simulink model "simulation_scheme_vel"  (R2021b)
settings: Solver=FixedStepAuto  StartTime=0.0  StopTime=simulation.stop_time  FixedStep=simulation.step_size  RelTol=1e-5
PreLoadFcn:
  | % initialize variables
  | initializeUnicycleModel;
undefined symbols (not defined in the file): camera, controller, obstacle, park, scheduler, simulation, tracking, unicycle
settings Model: Creator=beniamino  LastModifiedBy=gioel
settings SolverCC: AlgebraicLoopSolver=TrustRegion
settings DataIOCC: InitialState=cartesianInitialStates  SaveFormat=Structure

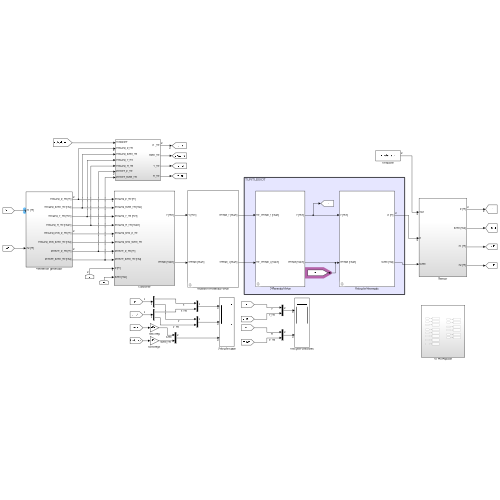
[thumbnail: Simulink's stored preview of the top-level diagram]
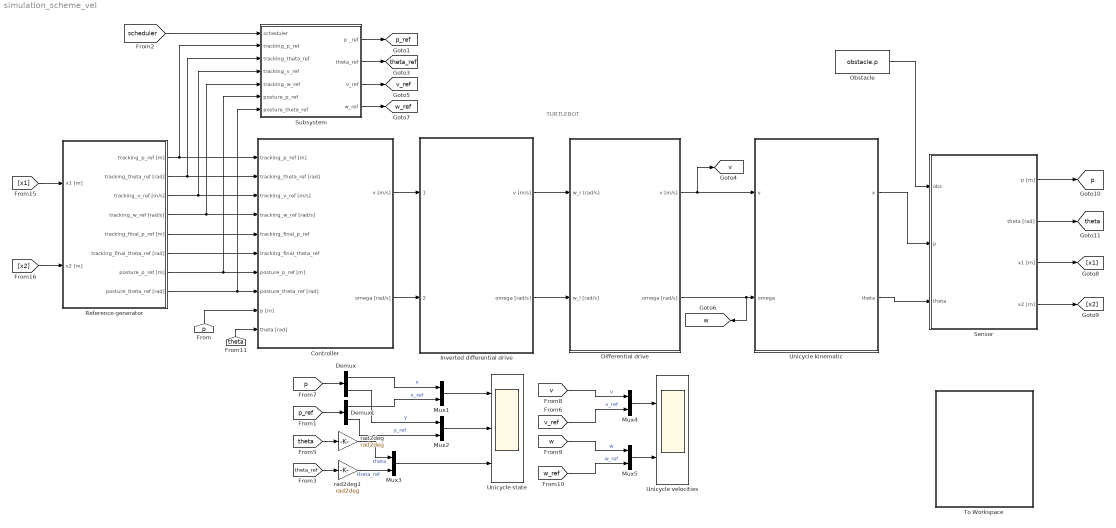
== system simulation_scheme_vel ==
  note: TURTLEBOT
  Controller : Subsystem
  Demux : Demux  Outputs=2
  Demux1 : Demux  Outputs=2
  Differential drive : Subsystem  mask(Differential drive for a unicycle){r=unicycle.diffDrive.r, d=unicycle.diffDrive.d, wheelDyEn=on, Tc=unicycle.diffDrive.Td, wheelsSpeedUpperLimit=unicycle.diffDrive.omegaWheelMax, wheelsSpeedLowerLimit=unicycle.diffDrive.omegaWheelMin}
      mask prompts: r "wheel radius"; d "interaxis lenght"; wheelDyEn "l.p.f. enable"; Tc "time constant [s]"; wheelsSpeedUpperLimit "max wheel speed  [rad/s]"; wheelsSpeedLowerLimit "min wheel speed [rad/s]"
      mask help:
      | Model of a differential drive.
      | It takes as input the derired wheel velocities and converts them to the corresponding driving velocity and stearing velocity.
      | Wheels dynamics can be taken into accont, along with output saturation.
      mask Help:
      | author: Beniamino Pozzan
      | email: beniamino.pozzan@phd.unipd.it
      mask Callback wheelDyEn:
      | % get the enable parameter
      | wheelDyEnStatus = get_param(gcb,'wheelDyEn');
      | enableStatus = get_param(gcb,'MaskEnables');
      | % if it is true, make Tc enabled
      | if strcmp(wheelDyEnStatus,'on')
      |     enableStatus{4}='on';
      | else
      |     enableStatus{4}='off';
      | end
      | set_param(gcb,'MaskEnables',enableStatus)
      mask TypeOptions wheelsSpeedUpperLimit: w_l saturator/UpperLimit | w_r saturator/UpperLimit
      mask TypeOptions wheelsSpeedLowerLimit: w_l saturator/LowerLimit | w_r saturator/LowerLimit
      mask DialogControl wheelDy Prompt: wheel dynamics
  Inverted differential drive : Subsystem  mask(Inverted Differential drive for a unicycle){r=unicycle.diffDrive.r, d=unicycle.diffDrive.d}
      mask prompts: r "wheel radius"; d "interaxis lenght"
      mask help:
      | Inverted differential drive for a unicycle.
      | Provided the desired driving and stearing velocities, it computes the corresponding wheel velocities.
  Mux{1..5} (5 alike) : Mux  Inputs=2
  Obstacle : Constant  Value=obstacle.p
  Reference generator : Subsystem
  Sensor : Subsystem
  Subsystem : Subsystem
  To Workspace : Subsystem
  Unicycle kinematic : Subsystem  mask(Unicycle Kinematic Model){x0=unicycle.ic.x, y0=unicycle.ic.y, theta0=unicycle.ic.theta}
      mask prompts: x0 "x_0"; y0 "y_0"; theta0 "theta_0"
      mask help: kinematic model of a unicyle.
  Unicycle state : Scope  NumInputPorts=3
  Unicycle velocities : Scope  NumInputPorts=2
  rad2deg : Gain  Gain=rad2deg
  rad2deg1 : Gain  Gain=rad2deg
  tag scope: p=global, p_ref=global, theta=global, theta_ref=global, v=global, v_ref=global, w=global, w_ref=global
  wires:
  Inverted differential drive/1(v [m/s]) -> Differential drive/1(w_r [rad/s])
  Inverted differential drive/2(omega [rad/s]) -> Differential drive/2(w_l [rad/s])
  Differential drive/1(v [m/s]) -> Unicycle kinematic/1(v), [v]
  Differential drive/2(omega [rad/s]) -> [w], Unicycle kinematic/2(omega)
  Unicycle kinematic/1(x) -> Sensor/2(p)
  Unicycle kinematic/2(theta) -> Sensor/3(theta)
  [p] -> Demux/1
  [p_ref] -> Demux1/1
  Mux1/1 -> Unicycle state/1
  Mux2/1 -> Unicycle state/2
  Demux/1 -> Mux1/1  "x"
  Demux1/1 -> Mux1/2  "x_ref"
  Demux/2 -> Mux2/1  "y"
  Demux1/2 -> Mux2/2  "y_ref"
  [theta_ref] -> rad2deg1/1
  Mux4/1 -> Unicycle velocities/1
  Mux5/1 -> Unicycle velocities/2
  [v] -> Mux4/1  "v"
  [v_ref] -> Mux4/2  "v_ref"
  [w] -> Mux5/1  "w"
  [w_ref] -> Mux5/2  "w_ref"
  [theta] -> Controller/10(theta [rad])
  Controller/1(v [m/s]) -> Inverted differential drive/1(1)
  Controller/2(omega [rad/s]) -> Inverted differential drive/2(2)
  Reference generator/1(tracking_p_ref [m]) -> Subsystem/2(tracking_p_ref), Controller/1(tracking_p_ref [m])
  Reference generator/4(tracking_w_ref [rad/s]) -> Subsystem/5(tracking_w_ref), Controller/4(tracking_w_ref [rad/s])
  Reference generator/2(tracking_theta_ref [rad]) -> Subsystem/3(tracking_theta_ref), Controller/2(tracking_theta_ref [rad])
  Reference generator/5(tracking_final_p_ref [m]) -> Controller/5(tracking_final_p_ref)
  Reference generator/6(tracking_final_theta_ref [rad]) -> Controller/6(tracking_final_theta_ref)
  Reference generator/7(posture_p_ref [m]) -> Subsystem/6(posture_p_ref), Controller/7(posture_p_ref [m])
  Reference generator/8(posture_theta_ref [rad]) -> Subsystem/7(posture_theta_ref), Controller/8(posture_theta_ref [rad])
  Reference generator/3(tracking_v_ref [m/s]) -> Subsystem/4(tracking_v_ref), Controller/3(tracking_v_ref [m/s])
  Mux3/1 -> Unicycle state/3
  Sensor/1(p [m]) -> [p]
  Sensor/2(theta [rad]) -> [theta]
  Sensor/3(x1 [m]) -> [x1]
  Sensor/4(x2 [m]) -> [x2]
  Obstacle/1 -> Sensor/1(obs)
  [x1] -> Reference generator/1(x1 [m])
  [x2] -> Reference generator/2(x2 [m])
  [p] -> Controller/9(p [m])
  [theta] -> rad2deg/1
  rad2deg/1 -> Mux3/1  "theta"
  rad2deg1/1 -> Mux3/2  "theta_ref"
  Subsystem/1(p _ref) -> [p_ref]
  Subsystem/2(theta_ref) -> [theta_ref]
  Subsystem/3(v_ref) -> [v_ref]
  Subsystem/4(w_ref) -> [w_ref]
  [scheduler] -> Subsystem/1(scheduler)

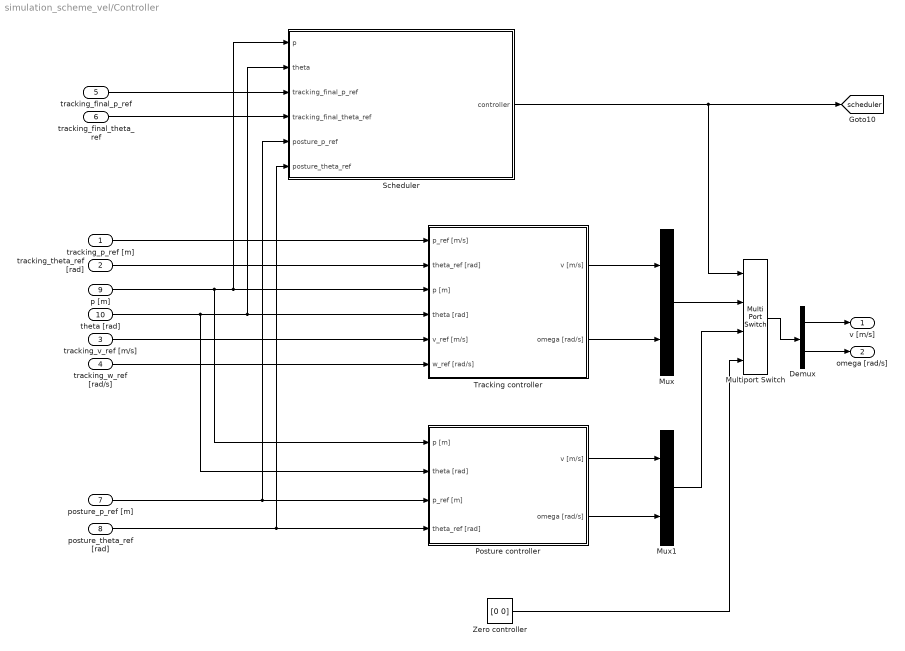
== system simulation_scheme_vel/Controller ==
  tracking_p_ref [m] : Inport
  tracking_theta_ref [rad] : Inport  Port=2
  tracking_v_ref [m/s] : Inport  Port=3
  tracking_w_ref [rad/s] : Inport  Port=4
  tracking_final_p_ref : Inport  Port=5
  tracking_final_theta_ref : Inport  Port=6
  posture_p_ref [m] : Inport  Port=7
  posture_theta_ref [rad] : Inport  Port=8
  p [m] : Inport  Port=9
  theta [rad] : Inport  Port=10
  Demux : Demux  Outputs=2
  Multiport Switch : MultiPortSwitch
  Mux : Mux  Inputs=2
  Mux1 : Mux  Inputs=2
  Posture controller : Subsystem
  Scheduler : MATLAB Function  TreatAsAtomicUnit=on
  Tracking controller : Subsystem
  Zero controller : Constant  Value=[0 0]
  v [m/s] : Outport
  omega [rad/s] : Outport  Port=2
  tag scope: scheduler=global
  wires:
  Multiport Switch/1 -> Demux/1
  Tracking controller/1(v [m/s]) -> Mux/1
  Tracking controller/2(omega [rad/s]) -> Mux/2
  Demux/2 -> omega [rad/s]/1
  Demux/1 -> v [m/s]/1
  Mux/1 -> Multiport Switch/2
  tracking_p_ref [m]/1 -> Tracking controller/1(p_ref [m/s])
  tracking_theta_ref [rad]/1 -> Tracking controller/2(theta_ref [rad])
  p [m]/1 -> Posture controller/1(p [m]), Tracking controller/3(p [m]), Scheduler/1(p)
  Zero controller/1 -> Multiport Switch/4
  Mux1/1 -> Multiport Switch/3
  Posture controller/2(omega [rad/s]) -> Mux1/2
  Posture controller/1(v [m/s]) -> Mux1/1
  Scheduler/1(controller) -> [scheduler], Multiport Switch/1
  theta [rad]/1 -> Posture controller/2(theta [rad]), Tracking controller/4(theta [rad]), Scheduler/2(theta)
  posture_p_ref [m]/1 -> Posture controller/3(p_ref [m]), Scheduler/5(posture_p_ref)
  posture_theta_ref [rad]/1 -> Scheduler/6(posture_theta_ref), Posture controller/4(theta_ref [rad])
  tracking_final_p_ref/1 -> Scheduler/3(tracking_final_p_ref)
  tracking_final_theta_ref/1 -> Scheduler/4(tracking_final_theta_ref)
  tracking_v_ref [m/s]/1 -> Tracking controller/5(v_ref [m/s])
  tracking_w_ref [rad/s]/1 -> Tracking controller/6(w_ref [rad/s])

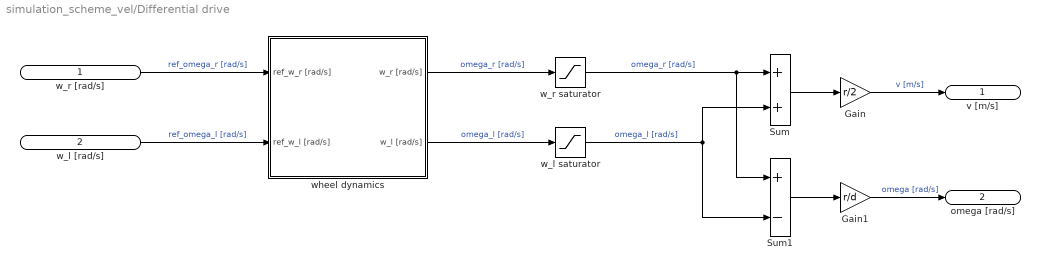
== system simulation_scheme_vel/Differential drive ==
  w_r [rad/s] : Inport  Unit=rad/s
  w_l [rad/s] : Inport  Port=2  Unit=rad/s
  Gain : Gain  Gain=r/2
  Gain1 : Gain  Gain=r/d
  Sum : Sum
  Sum1 : Sum  Inputs=+-
  w_l saturator : Saturate  UpperLimit=wheelsSpeedUpperLimit  LowerLimit=wheelsSpeedLowerLimit
  w_r saturator : Saturate  UpperLimit=wheelsSpeedUpperLimit  LowerLimit=wheelsSpeedLowerLimit
  wheel dynamics : Subsystem  Variant=on
  v [m/s] : Outport  Unit=m/s
  omega [rad/s] : Outport  Port=2  Unit=rad/s
  wires:
  w_l saturator/1 -> Sum1/2, Sum/2  "omega_l [rad/s]"
  w_r saturator/1 -> Sum1/1, Sum/1  "omega_r [rad/s]"
  Gain1/1 -> omega [rad/s]/1  "omega [rad/s]"
  Sum1/1 -> Gain1/1
  Gain/1 -> v [m/s]/1  "v [m/s]"
  Sum/1 -> Gain/1
  w_r [rad/s]/1 -> wheel dynamics/1(ref_w_r [rad/s])  "ref_omega_r [rad/s]"
  w_l [rad/s]/1 -> wheel dynamics/2(ref_w_l [rad/s])  "ref_omega_l [rad/s]"
  wheel dynamics/1(w_r [rad/s]) -> w_r saturator/1  "omega_r [rad/s]"
  wheel dynamics/2(w_l [rad/s]) -> w_l saturator/1  "omega_l [rad/s]"

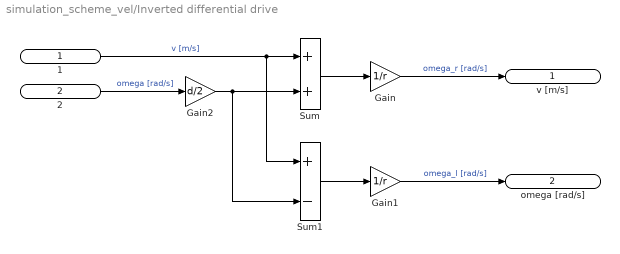
== system simulation_scheme_vel/Inverted differential drive ==
  1 : Inport  Unit=m/s
  2 : Inport  Port=2  Unit=rad/s
  Gain : Gain  Gain=1/r
  Gain1 : Gain  Gain=1/r
  Gain2 : Gain  Gain=d/2
  Sum : Sum
  Sum1 : Sum  Inputs=+-
  v [m/s] : Outport  Unit=rad/s
  omega [rad/s] : Outport  Port=2  Unit=rad/s
  wires:
  Gain2/1 -> Sum1/2, Sum/2
  Sum/1 -> Gain/1
  Gain/1 -> v [m/s]/1  "omega_r [rad/s]"
  Sum1/1 -> Gain1/1
  Gain1/1 -> omega [rad/s]/1  "omega_l [rad/s]"
  1/1 -> Sum1/1, Sum/1  "v [m/s]"
  2/1 -> Gain2/1  "omega [rad/s]"

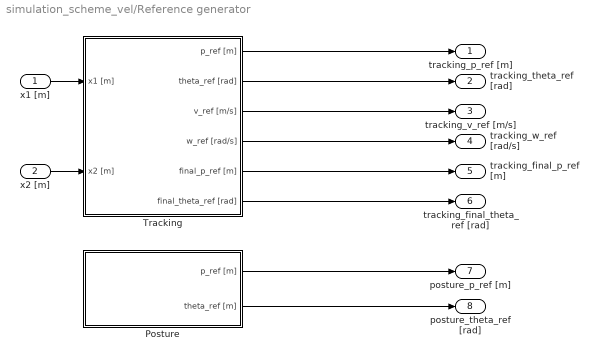
== system simulation_scheme_vel/Reference generator ==
  x1 [m] : Inport
  x2 [m] : Inport  Port=2
  Posture : Subsystem
  Tracking : Subsystem
  tracking_p_ref [m] : Outport
  tracking_theta_ref [rad] : Outport  Port=2
  tracking_v_ref [m/s] : Outport  Port=3
  tracking_w_ref [rad/s] : Outport  Port=4
  tracking_final_p_ref [m] : Outport  Port=5
  tracking_final_theta_ref [rad] : Outport  Port=6
  posture_p_ref [m] : Outport  Port=7
  posture_theta_ref [rad] : Outport  Port=8
  wires:
  Tracking/4(w_ref [rad/s]) -> tracking_w_ref [rad/s]/1
  Tracking/3(v_ref [m/s]) -> tracking_v_ref [m/s]/1
  Posture/1(p_ref [m]) -> posture_p_ref [m]/1
  Tracking/5(final_p_ref [m]) -> tracking_final_p_ref [m]/1
  Tracking/2(theta_ref [rad]) -> tracking_theta_ref [rad]/1
  Tracking/6(final_theta_ref [rad]) -> tracking_final_theta_ref [rad]/1
  Tracking/1(p_ref [m]) -> tracking_p_ref [m]/1
  Posture/2(theta_ref [m]) -> posture_theta_ref [rad]/1
  x2 [m]/1 -> Tracking/2(x2 [m])
  x1 [m]/1 -> Tracking/1(x1 [m])

== system simulation_scheme_vel/Sensor ==
  obs : Inport
  p : Inport  Port=2
  theta : Inport  Port=3
  Demux : Demux  Outputs=2
  camera : MATLAB Function  TreatAsAtomicUnit=on
  p [m] : Outport
  theta [rad] : Outport  Port=2
  x1 [m] : Outport  Port=3
  x2 [m] : Outport  Port=4
  wires:
  camera/2(x2) -> x2 [m]/1
  camera/1(x1) -> x1 [m]/1
  theta/1 -> camera/3(theta), theta [rad]/1
  obs/1 -> camera/4(obs_W)
  p/1 -> Demux/1, p [m]/1
  Demux/1 -> camera/1(x_pos)
  Demux/2 -> camera/2(y_pos)

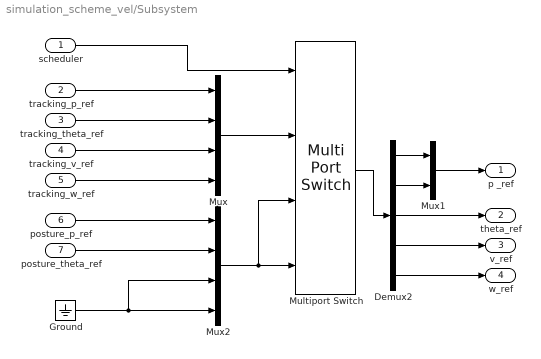
== system simulation_scheme_vel/Subsystem ==
  scheduler : Inport
  tracking_p_ref : Inport  Port=2
  tracking_theta_ref : Inport  Port=3
  tracking_v_ref : Inport  Port=4
  tracking_w_ref : Inport  Port=5
  posture_p_ref : Inport  Port=6
  posture_theta_ref : Inport  Port=7
  Demux2 : Demux  Outputs=5
  Ground : Ground
  Multiport Switch : MultiPortSwitch
  Mux : Mux
  Mux1 : Mux  Inputs=2
  Mux2 : Mux
  p _ref : Outport
  theta_ref : Outport  Port=2
  v_ref : Outport  Port=3
  w_ref : Outport  Port=4
  wires:
  tracking_theta_ref/1 -> Mux/2
  scheduler/1 -> Multiport Switch/1
  tracking_p_ref/1 -> Mux/1
  Multiport Switch/1 -> Demux2/1
  Mux/1 -> Multiport Switch/2
  Ground/1 -> Mux2/3, Mux2/4
  tracking_v_ref/1 -> Mux/3
  tracking_w_ref/1 -> Mux/4
  Mux2/1 -> Multiport Switch/3, Multiport Switch/4
  posture_p_ref/1 -> Mux2/1
  posture_theta_ref/1 -> Mux2/2
  Demux2/1 -> Mux1/1
  Demux2/2 -> Mux1/2
  Mux1/1 -> p _ref/1
  Demux2/3 -> theta_ref/1
  Demux2/4 -> v_ref/1
  Demux2/5 -> w_ref/1

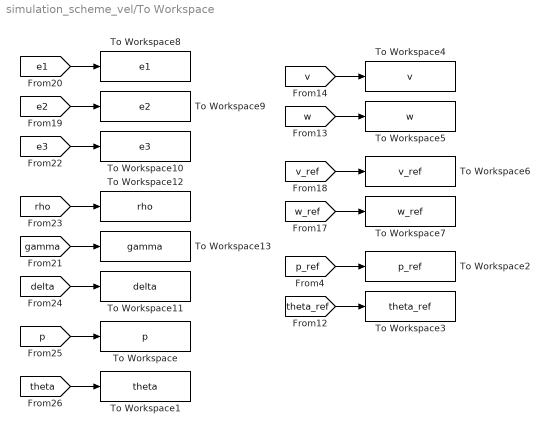
== system simulation_scheme_vel/To Workspace ==
  To Workspace : ToWorkspace  VariableName=p  SaveFormat=Timeseries  SampleTime=-1
  To Workspace1 : ToWorkspace  VariableName=theta  SaveFormat=Timeseries  SampleTime=-1
  To Workspace10 : ToWorkspace  VariableName=e3  SaveFormat=Timeseries  SampleTime=-1
  To Workspace11 : ToWorkspace  VariableName=delta  SaveFormat=Timeseries  SampleTime=-1
  To Workspace12 : ToWorkspace  VariableName=rho  SaveFormat=Timeseries  SampleTime=-1
  To Workspace13 : ToWorkspace  VariableName=gamma  SaveFormat=Timeseries  SampleTime=-1
  To Workspace2 : ToWorkspace  VariableName=p_ref  SaveFormat=Timeseries  SampleTime=-1
  To Workspace3 : ToWorkspace  VariableName=theta_ref  SaveFormat=Timeseries  SampleTime=-1
  To Workspace4 : ToWorkspace  VariableName=v  SaveFormat=Timeseries  SampleTime=-1
  To Workspace5 : ToWorkspace  VariableName=w  SaveFormat=Timeseries  SampleTime=-1
  To Workspace6 : ToWorkspace  VariableName=v_ref  SaveFormat=Timeseries  SampleTime=-1
  To Workspace7 : ToWorkspace  VariableName=w_ref  SaveFormat=Timeseries  SampleTime=-1
  To Workspace8 : ToWorkspace  VariableName=e1  SaveFormat=Timeseries  SampleTime=-1
  To Workspace9 : ToWorkspace  VariableName=e2  SaveFormat=Timeseries  SampleTime=-1
  wires:
  [v_ref] -> To Workspace6/1
  [w_ref] -> To Workspace7/1
  [theta] -> To Workspace1/1
  [e1] -> To Workspace8/1
  [v] -> To Workspace4/1
  [e2] -> To Workspace9/1
  [delta] -> To Workspace11/1
  [gamma] -> To Workspace13/1
  [e3] -> To Workspace10/1
  [w] -> To Workspace5/1
  [rho] -> To Workspace12/1
  [p_ref] -> To Workspace2/1
  [theta_ref] -> To Workspace3/1
  [p] -> To Workspace/1

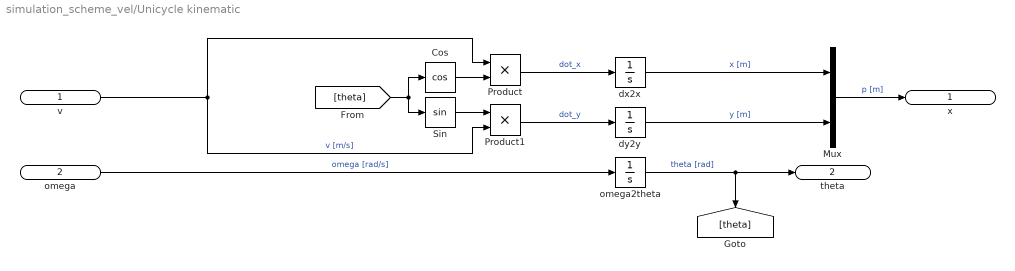
== system simulation_scheme_vel/Unicycle kinematic ==
  v : Inport  PortDimensions=1
  omega : Inport  Port=2  PortDimensions=1
  Cos : Trigonometry  Operator=cos
  Mux : Mux  Inputs=2
  Product : Product
  Product1 : Product
  Sin : Trigonometry
  dx2x : Integrator  InitialCondition=x0  ContinuousStateAttributes='pos_x'
  dy2y : Integrator  InitialCondition=y0  ContinuousStateAttributes='pos_y'
  omega2theta : Integrator  InitialCondition=theta0  ContinuousStateAttributes='theta'
  x : Outport  PortDimensions=2
  theta : Outport  Port=2  PortDimensions=1
  wires:
  Product1/1 -> dy2y/1  "dot_y"
  [theta] -> Sin/1, Cos/1
  v/1 -> Product/1, Product1/2  "v [m/s]"
  omega2theta/1 -> [theta], theta/1  "theta [rad]"
  omega/1 -> omega2theta/1  "omega [rad/s]"
  dy2y/1 -> Mux/2  "y [m]"
  Cos/1 -> Product/2
  dx2x/1 -> Mux/1  "x [m]"
  Sin/1 -> Product1/1
  Product/1 -> dx2x/1  "dot_x"
  Mux/1 -> x/1  "p [m]"

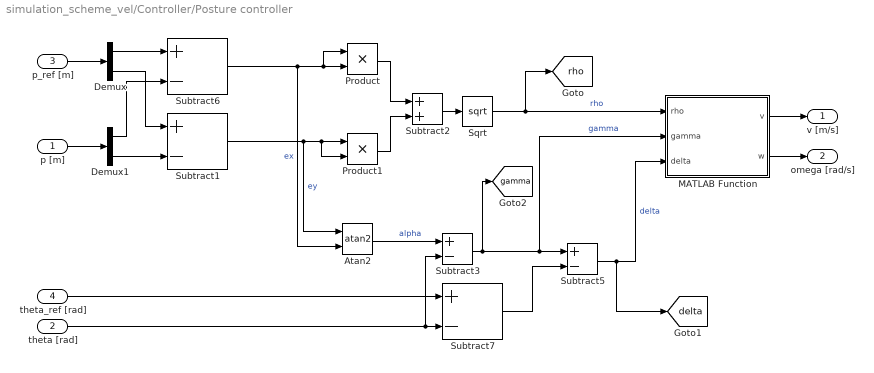
== system simulation_scheme_vel/Controller/Posture controller ==
  p [m] : Inport
  theta [rad] : Inport  Port=2
  p_ref [m] : Inport  Port=3
  theta_ref [rad] : Inport  Port=4
  Atan2 : Trigonometry  Operator=atan2
  Demux : Demux  Outputs=2
  Demux1 : Demux  Outputs=2
  MATLAB Function : MATLAB Function  TreatAsAtomicUnit=on
  Product : Product
  Product1 : Product
  Sqrt : Sqrt  SaturateOnIntegerOverflow=on
  Subtract{1,3,5..7} (5 alike) : Sum  Inputs=+-
  Subtract2 : Sum
  v [m/s] : Outport
  omega [rad/s] : Outport  Port=2
  tag scope: delta=global, gamma=global, rho=global
  wires:
  p_ref [m]/1 -> Demux/1
  p [m]/1 -> Demux1/1
  Subtract6/1 -> Atan2/2, Product/1, Product/2  "ex"
  Subtract1/1 -> Product1/1, Product1/2, Atan2/1  "ey"
  Product1/1 -> Subtract2/2
  Product/1 -> Subtract2/1
  Subtract2/1 -> Sqrt/1
  Sqrt/1 -> [rho], MATLAB Function/1(rho)  "rho"
  Subtract3/1 -> [gamma], Subtract5/1, MATLAB Function/2(gamma)  "gamma"
  theta [rad]/1 -> Subtract7/2, Subtract3/2
  MATLAB Function/1(v) -> v [m/s]/1
  MATLAB Function/2(w) -> omega [rad/s]/1
  Subtract5/1 -> [delta], MATLAB Function/3(delta)  "delta"
  Atan2/1 -> Subtract3/1  "alpha"
  Demux/1 -> Subtract6/1
  Demux1/1 -> Subtract6/2
  Demux/2 -> Subtract1/1
  Demux1/2 -> Subtract1/2
  theta_ref [rad]/1 -> Subtract7/1
  Subtract7/1 -> Subtract5/2

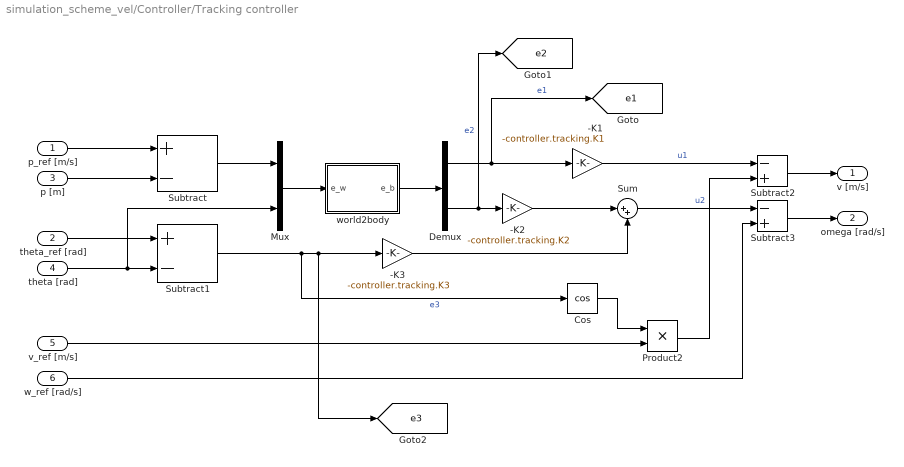
== system simulation_scheme_vel/Controller/Tracking controller ==
  p_ref [m/s] : Inport
  theta_ref [rad] : Inport  Port=2
  p [m] : Inport  Port=3
  theta [rad] : Inport  Port=4
  v_ref [m/s] : Inport  Port=5
  w_ref [rad/s] : Inport  Port=6
  -K1 : Gain  Gain=-controller.tracking.K1
  -K2 : Gain  Gain=-controller.tracking.K2
  -K3 : Gain  Gain=-controller.tracking.K3
  Cos : Trigonometry  Operator=cos
  Demux : Demux  Outputs=2
  Mux : Mux  Inputs=2
  Product2 : Product
  Subtract : Sum  Inputs=+-
  Subtract1 : Sum  Inputs=+-
  Subtract2 : Sum  Inputs=-+
  Subtract3 : Sum  Inputs=-+
  Sum : Sum  Inputs=|++
  world2body : MATLAB Function  TreatAsAtomicUnit=on
  v [m/s] : Outport
  omega [rad/s] : Outport  Port=2
  tag scope: e1=global, e2=global, e3=global
  wires:
  Subtract2/1 -> v [m/s]/1
  -K1/1 -> Subtract2/1  "u1"
  theta [rad]/1 -> Mux/2, Subtract1/2
  p [m]/1 -> Subtract/2
  Subtract/1 -> Mux/1
  Demux/2 -> [e2], -K2/1  "e2"
  -K2/1 -> Sum/1
  Subtract3/1 -> omega [rad/s]/1
  Mux/1 -> world2body/1(e_w)
  Cos/1 -> Product2/1
  theta_ref [rad]/1 -> Subtract1/1
  -K3/1 -> Sum/2
  Sum/1 -> Subtract3/1  "u2"
  Demux/1 -> [e1], -K1/1  "e1"
  Product2/1 -> Subtract2/2
  world2body/1(e_b) -> Demux/1
  Subtract1/1 -> Cos/1, -K3/1, [e3]  "e3"
  p_ref [m/s]/1 -> Subtract/1
  v_ref [m/s]/1 -> Product2/2
  w_ref [rad/s]/1 -> Subtract3/2

== system simulation_scheme_vel/Differential drive/wheel dynamics ==
  ref_w_r [rad/s] : Inport
  ref_w_l [rad/s] : Inport  Port=2
  lpf : Subsystem  VariantControl=wheelDyEn==true
  none : Subsystem  VariantControl=wheelDyEn==false
  w_r [rad/s] : Outport
  w_l [rad/s] : Outport  Port=2

== system simulation_scheme_vel/Reference generator/Posture ==
  Constant : Constant  Value=park.y  SampleTime=unicycle.diffDrive.Td
  Constant1 : Constant  Value=park.x  SampleTime=unicycle.diffDrive.Td
  Constant2 : Constant  Value=park.theta  SampleTime=unicycle.diffDrive.Td
  Mux : Mux  Inputs=2
  p_ref [m] : Outport
  theta_ref [m] : Outport  Port=2
  wires:
  Mux/1 -> p_ref [m]/1
  Constant1/1 -> Mux/1
  Constant/1 -> Mux/2
  Constant2/1 -> theta_ref [m]/1

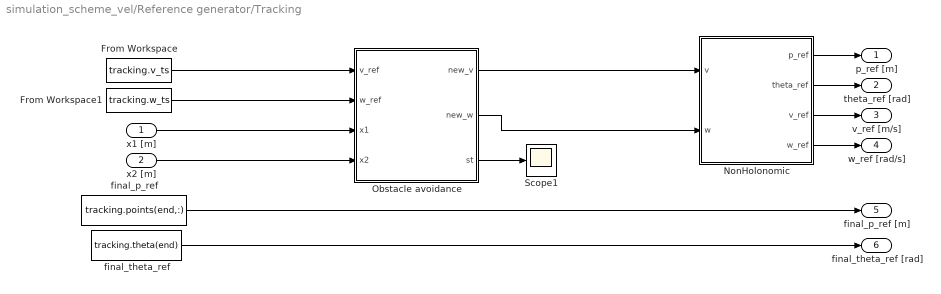
== system simulation_scheme_vel/Reference generator/Tracking ==
  x1 [m] : Inport
  x2 [m] : Inport  Port=2
  From Workspace : FromWorkspace  VariableName=tracking.v_ts  SampleTime=unicycle.diffDrive.Td
  From Workspace1 : FromWorkspace  VariableName=tracking.w_ts  SampleTime=unicycle.diffDrive.Td
  NonHolonomic : Subsystem
  Obstacle avoidance : MATLAB Function  TreatAsAtomicUnit=on
  Scope1 : Scope
  final_p_ref : Constant  Value=tracking.points(end,:)
  final_theta_ref : Constant  Value=tracking.theta(end)
  p_ref [m] : Outport
  theta_ref [rad] : Outport  Port=2
  v_ref [m/s] : Outport  Port=3
  w_ref [rad/s] : Outport  Port=4
  final_p_ref [m] : Outport  Port=5
  final_theta_ref [rad] : Outport  Port=6
  wires:
  final_p_ref/1 -> final_p_ref [m]/1
  final_theta_ref/1 -> final_theta_ref [rad]/1
  NonHolonomic/3(v_ref) -> v_ref [m/s]/1
  NonHolonomic/1(p_ref) -> p_ref [m]/1
  NonHolonomic/4(w_ref) -> w_ref [rad/s]/1
  NonHolonomic/2(theta_ref) -> theta_ref [rad]/1
  x1 [m]/1 -> Obstacle avoidance/3(x1)
  x2 [m]/1 -> Obstacle avoidance/4(x2)
  From Workspace/1 -> Obstacle avoidance/1(v_ref)
  From Workspace1/1 -> Obstacle avoidance/2(w_ref)
  Obstacle avoidance/3(st) -> Scope1/1
  Obstacle avoidance/1(new_v) -> NonHolonomic/1(v)
  Obstacle avoidance/2(new_w) -> NonHolonomic/2(w)

== system simulation_scheme_vel/Differential drive/wheel dynamics/lpf ==
  ref_w_r [rad/s] : Inport
  ref_w_l [rad/s] : Inport  Port=2
  w_r_lpf : TransferFcn  Denominator=[Tc 1]  ContinuousStateAttributes='w_r_lpf'
  w_r_lpf1 : TransferFcn  Denominator=[Tc 1]  ContinuousStateAttributes='w_r_lpf'
  w_r [rad/s] : Outport
  w_l [rad/s] : Outport  Port=2
  wires:
  ref_w_r [rad/s]/1 -> w_r_lpf/1
  w_r_lpf1/1 -> w_l [rad/s]/1  "w_r [rad/s]"
  w_r_lpf/1 -> w_r [rad/s]/1  "w_l [rad/s]"
  ref_w_l [rad/s]/1 -> w_r_lpf1/1  "w_r [rad/s]"

== system simulation_scheme_vel/Differential drive/wheel dynamics/none ==
  ref_w_r [rad/s] : Inport
  ref_w_l [rad/s] : Inport  Port=2
  w_r [rad/s] : Outport
  w_l [rad/s] : Outport  Port=2
  wires:
  ref_w_r [rad/s]/1 -> w_r [rad/s]/1  "w_l [rad/s]"
  ref_w_l [rad/s]/1 -> w_l [rad/s]/1  "w_r [rad/s]"

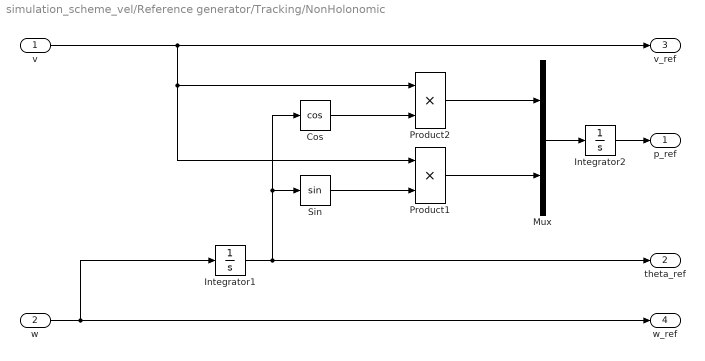
== system simulation_scheme_vel/Reference generator/Tracking/NonHolonomic ==
  v : Inport
  w : Inport  Port=2
  Cos : Trigonometry  Operator=cos
  Integrator1 : Integrator  InitialCondition=tracking.theta0
  Integrator2 : Integrator  InitialCondition=[tracking.x0 tracking.y0]
  Mux : Mux  Inputs=2
  Product1 : Product
  Product2 : Product
  Sin : Trigonometry
  p_ref : Outport
  theta_ref : Outport  Port=2
  v_ref : Outport  Port=3
  w_ref : Outport  Port=4
  wires:
  Integrator2/1 -> p_ref/1
  Mux/1 -> Integrator2/1
  Product1/1 -> Mux/2
  Product2/1 -> Mux/1
  v/1 -> Product2/1, Product1/1, v_ref/1
  Integrator1/1 -> theta_ref/1, Sin/1, Cos/1
  w/1 -> Integrator1/1, w_ref/1
  Cos/1 -> Product2/2
  Sin/1 -> Product1/2

== matlab function simulation_scheme_vel/Controller/Tracking controller/world2body ==
  data: e_w input; e_b output
function e_b = fcn(e_w)

%
% This function expresses the position and orientation error wrt RF_B
%
% Inputs:
% e_w    : e_w = [e_x; e_y; e_theta] wrt RF_W
%
% Outputs:
% e_b    : e_b = [e_x; e_y; e_theta] wrt RF_B

e_b = [cos(e_w(3)) sin(e_w(3)); -sin(e_w(3)) cos(e_w(3))] * [e_w(1); e_w(2)];

== matlab function simulation_scheme_vel/Controller/Scheduler ==
  settings: updateMethod=DISCRETE  sampleTime=unicycle.diffDrive.Td
  data: p input; theta input; controller output; tracking_final_p_ref input; tracking_final_theta_ref input; posture_p_ref input; posture_theta_ref input; simulation parameter; scheduler parameter
function controller  =  fcn(p, theta, tracking_final_p_ref, tracking_final_theta_ref, ...
      posture_p_ref, posture_theta_ref, simulation, scheduler)

%
% This function returns the index of the active controller
% (tracking controller , posture controller, no controller)
%
% Inputs:
% p                        : current position of the agent
% theta                    : current orientation of the agent
% tracking_final_p_ref     : final tracking reference position
% tracking_final_theta_ref : final tracking reference orientation
% posture_p_ref            : parking place position
% posture_theta_ref        : parking place orientation
%
% Outputs:
% controller               : index of the active controller

% State: index of the active controller
% 1 - tracking controller
% 2 - posture controller
% 3 - zero controller
persistent state;

% inizialition
if isempty(state)

   state = simulation.starting_controller;
end

switch state
    case 1

        % Check if the agent reaches the end of the track
        if (norm(p-tracking_final_p_ref) <= scheduler.threshold_p) && ...
           (abs(theta-tracking_final_theta_ref) <= scheduler.threshold_theta)
            state = 2;
        end
    
    case 2

        % Check if the agent reaches the desired position
        if (norm(p-posture_p_ref) <= scheduler.threshold_p) && ...
           (abs(theta-posture_theta_ref) <= scheduler.threshold_theta) 
            state = 3;
        end
    
    case 3

        % Do nothing
end

% Return the index of the active controller
controller = state;

end

== matlab function simulation_scheme_vel/Controller/Posture controller/MATLAB Function ==
  data: rho input; gamma input; delta input; v output; w output; controller parameter
function [v,w] = fcn(rho, gamma, delta, controller)

%
% This function computes the feedback control law acting on v, w
%
% Inputs:
% rho   : length of the error vector
% delta : atan2(y_pos, x_pos) + pi
% gamma : delta - theta
%
% Outputs:
% v     : linear velocity
% w     : angular velocity

v = controller.posture.Kv * rho * cos(gamma);
w = controller.posture.Kw * gamma + controller.posture.Kv * ... 
    sin(gamma) * cos(gamma) / gamma * (gamma + ...
    controller.posture.Kdelta * delta);

== matlab function simulation_scheme_vel/Sensor/camera ==
  settings: updateMethod=DISCRETE  sampleTime=0.01
  data: x_pos input; x1 output; x2 output; y_pos input; theta input; obs_W input; camera parameter; unicycle parameter
 function [x1, x2] = fcn(x_pos, y_pos, theta, obs_W, camera, unicycle)

%
% Inputs
% x_pos: x coordinate of the agent wrt RF_W
% y_pos: y coordinate of the agent wrt RF_W
% theta: orientation of the agent
% obs_W: position of the obstacle wrt RF_W
%
% Outputs
% x1: Camera1 image plane coordinate
% x2: Camera2 image plane coordinate

% Rotation matrix definition
R_WB = [cos(theta) -sin(theta); sin(theta) cos(theta)]; % Body to World
R_CW = transpose(R_WB*unicycle.R_BC); % World to Camera

% Translation matrix definition
T_WB = [x_pos;y_pos];

% Express obstacle in C1,C2 RFs
obs_C1 = R_CW*obs_W - transpose(unicycle.R_BC)*unicycle.T_BC1 - R_CW*T_WB;
obs_C2 = R_CW*obs_W - transpose(unicycle.R_BC)*unicycle.T_BC2 - R_CW*T_WB;

if obs_C1(2) > camera.focal_length && norm(obs_C1) < camera.depth && ...
   atan2(obs_C1(2), obs_C1(1)) >= - camera.fov && ...
   atan2(obs_C1(2), obs_C1(1)) <= camera.fov
   % Obstacle in C1 image plane
   x1 = camera.focal_length*(obs_C1(1)/obs_C1(2));
else
   x1 = nan;
end
if obs_C2(2) > camera.focal_length && norm(obs_C2) < camera.depth && ...
   atan2(obs_C2(2), obs_C2(1)) >= - camera.fov && ...
   atan2(obs_C2(2), obs_C2(1)) <= camera.fov
   % Obstacle in C2 image plane
   x2 = camera.focal_length*(obs_C2(1)/obs_C2(2));
else
   x2 = nan;
end

== matlab function simulation_scheme_vel/Reference generator/Tracking/Obstacle avoidance ==
  settings: updateMethod=DISCRETE  sampleTime=0.001
  data: v_ref input; w_ref input; x1 input; new_v output; new_w output; x2 input; st output; camera parameter; unicycle parameter; simulation parameter
function [new_v, new_w, st]   = fcn(v_ref, w_ref, x1, x2, camera, unicycle, simulation)

%
% The following obstacle avoidance method works only when starting point and
% final point of the overcoming procedure are placed in the same straight line
% The agent overcomes the obstacle by steering always first to the left
%
% Inputs:
% v_ref   : original reference linear velocity signal 
% w_ref   : original reference angular velocity signal 
% x1      : camera1 image plane coordinate
% x2      : camera2 image plane coordinate
%
% Outputs:
% new_v   : new reference linear velocity signal 
% new_w   : new reference angular velocity signal 
% st      : state

% state = 0 --> Agent is following original tracking trajectory
% state = 1 --> Agent is following first predefined curvilinear stretch
% state = 2 --> Agent is following second predefined curvilinear stretch
% state = 3 --> Agent is following third predefined straight stretch
% state = 4 --> Agent is following fourth predefined curvilinear stretch
% state = 5 --> Agent is following fifth predefined curvilinear stretch
persistent state

% Count instants for each state
persistent count

% Necessary to define the overcoming manouver
steering_radius = 0.25;
persistent steering_tang_vel
persistent steering_duration
persistent overcoming_length

% Initialize persistent variables
if isempty(state)
    state = 0;
    count = 0;
    steering_radius = 0;
    steering_tang_vel = 0;
    steering_duration = 0;
    overcoming_length = 0;

end

% steering_radius = 0.25; % Steering radius
% overcoming_length = 0.8; % Overcoming length (straight line)
% %overcoming_length = 2 * (unicycle.dangeroud_distance - 2*steering_radius);
% total_length = 2 * pi * steering_radius + overcoming_length; % Total length (straigth line + curvilinear stretches)
% reference_length = 4 * steering_radius + overcoming_length; % Reference length
% reference_duration = reference_length / v_ref; % Reference duration
% % Tangential velocity s.t. 
% % duration of the ovecoming procedure = duration original tracking
% steering_tang_vel = total_length / reference_duration;
% % Duration of 1 curvilinear stretch
% steering_duration = 0.5 * pi * steering_radius / steering_tang_vel; %[s]

switch state
    case 0
        % Mantain the reference velocities
        new_v = v_ref;
        new_w = w_ref;
        
        % Detect the obstacle and check if it is too near
        if(not(isnan(x1)) && not(isnan(x2)))
           
            % Triangulation
            py_C1 = unicycle.b*camera.focal_length/(x1 - x2); % y coordinate in RF_C1
            px_C1 = x1*unicycle.b/(x1 - x2); % x coordinate in RF_C1
            
            % If the obstacle is too near, start the overcoming procedure
            if py_C1 > camera.focal_length && py_C1 <= unicycle.dangerous_distance


                steering_radius = 0.25; % Steering radius
                overcoming_length = 2 * (py_C1 - 2*steering_radius);
                total_length = 2 * pi * steering_radius + overcoming_length; % Total length (straigth line + curvilinear stretches)
                reference_length = 4 * steering_radius + overcoming_length; % Reference length
                reference_duration = reference_length / v_ref; % Reference duration
                % Tangential velocity s.t. 
                % duration of the ovecoming procedure = duration original tracking
                steering_tang_vel = total_length / reference_duration;
                % Duration of 1 curvilinear stretch
                steering_duration = 0.5 * pi * steering_radius / steering_tang_vel; %[s]

                state = 1;
                count = 0;
            end
        end

    case 1
        count = count + 1;
        new_v = steering_tang_vel; 
        new_w = new_v / steering_radius; % Steer to the left

        if count >= steering_duration / simulation.step_size
            state = 2;
            count = 0;
        end
        
    case 2
       count = count + 1;
       new_v = steering_tang_vel; 
       new_w = - new_v / steering_radius; % Steer to the right

        if count >= steering_duration / simulation.step_size
            state = 3;
            count = 0;
        end

    case 3
        count = count + 1;
        new_v = steering_tang_vel; 
        new_w = 0; % Stop steering

        if count >= (overcoming_length/steering_tang_vel) / simulation.step_size
            state = 4;
            count = 0;
        end

    case 4
        count = count + 1;
        new_v = steering_tang_vel;
        new_w = - new_v / steering_radius; % Steer to the right

        if count >= steering_duration / simulation.step_size
            state = 5;
            count = 0;
        end

    case 5
        count = count + 1;
        new_v = steering_tang_vel;
        new_w = new_v / steering_radius; % Steer to the left

        if count >= steering_duration / simulation.step_size 
            state = 0;
            count = 0;
        end
    
    otherwise
        new_v = v_ref;
        new_w = w_ref;
end

st = state;
